simulink model "P2"  (R2020b)
settings: Solver=VariableStepAuto  StartTime=0.0  StopTime=10.0  RelTol=1e-3
settings Model: Creator=stank  LastModifiedBy=stank

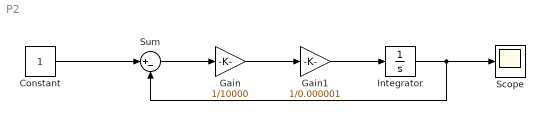
== system P2 ==
  Constant : Constant
  Gain : Gain  Gain=1/10000
  Gain1 : Gain  Gain=1/0.000001
  Integrator : Integrator
  Scope : Scope
  Sum : Sum  Inputs=|+-
  wires:
  Gain1/1 -> Integrator/1
  Integrator/1 -> Sum/2, Scope/1
  Sum/1 -> Gain/1
  Constant/1 -> Sum/1
  Gain/1 -> Gain1/1
